simulink model "labFinal_6"  (R2018b)
settings: Solver=FixedStepDiscrete  StartTime=0.0  StopTime=10.0  FixedStep=1  RelTol=1e-3
libraries: hdlsllib x49
settings Model: Creator=mllax8  LastModifiedBy=mllax8

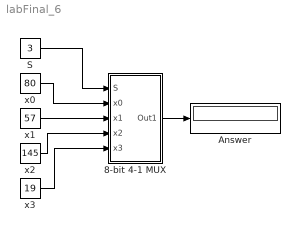
== system labFinal_6 ==
  8-bit 4-1 MUX : Subsystem
  Answer : Display
  S : Constant  Value=3  OutDataTypeStr=uint8  SampleTime=1
  x0 : Constant  Value=80  OutDataTypeStr=uint8  SampleTime=1
  x1 : Constant  Value=57  OutDataTypeStr=uint8  SampleTime=1
  x2 : Constant  Value=145  OutDataTypeStr=uint8  SampleTime=1
  x3 : Constant  Value=19  OutDataTypeStr=uint8  SampleTime=1
  wires:
  x0/1 -> 8-bit 4-1 MUX/2(x0)
  x1/1 -> 8-bit 4-1 MUX/3(x1)
  x2/1 -> 8-bit 4-1 MUX/4(x2)
  x3/1 -> 8-bit 4-1 MUX/5(x3)
  8-bit 4-1 MUX/1(Out1) -> Answer/1
  S/1 -> 8-bit 4-1 MUX/1(S)

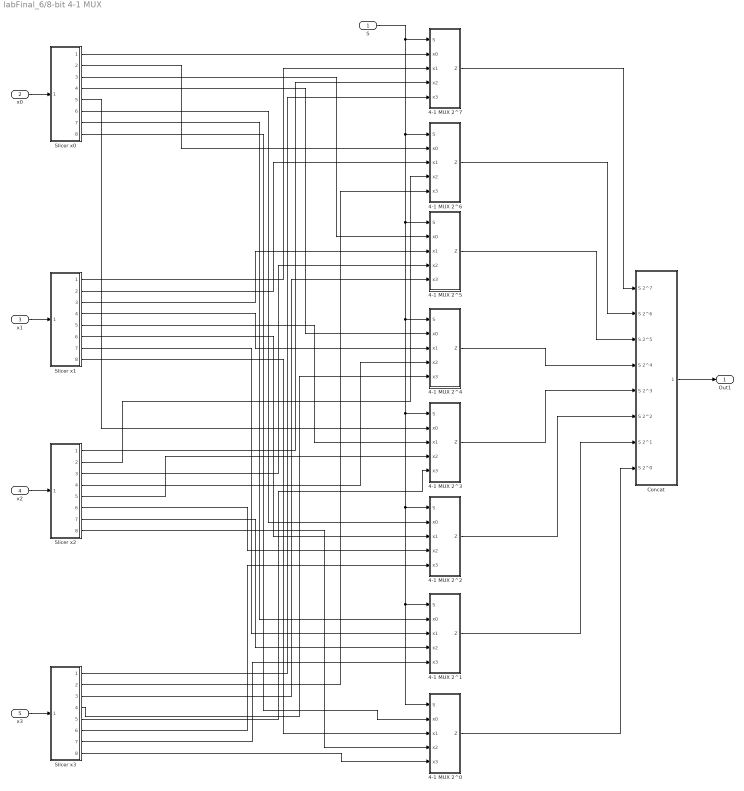
== system labFinal_6/8-bit 4-1 MUX ==
  S : Inport
  x0 : Inport  Port=2
  x1 : Inport  Port=3
  x2 : Inport  Port=4
  x3 : Inport  Port=5
  4-1 MUX 2^0 : Subsystem
  4-1 MUX 2^1 : Subsystem
  4-1 MUX 2^2 : Subsystem
  4-1 MUX 2^3 : Subsystem
  4-1 MUX 2^4 : Subsystem
  4-1 MUX 2^5 : Subsystem
  4-1 MUX 2^6 : Subsystem
  4-1 MUX 2^7 : Subsystem
  Concat : Subsystem
  Slicer x0 : Subsystem
  Slicer x1 : Subsystem
  Slicer x2 : Subsystem
  Slicer x3 : Subsystem
  Out1 : Outport
  wires:
  x1/1 -> Slicer x1/1(uint8)
  x0/1 -> Slicer x0/1(uint8)
  4-1 MUX 2^0/1(Z) -> Concat/8(S 2^0)
  Slicer x2/2(B 2^6) -> 4-1 MUX 2^6/4(x2)
  4-1 MUX 2^2/1(Z) -> Concat/6(S 2^2)
  Slicer x2/7(B 2^1) -> 4-1 MUX 2^1/4(x2)
  4-1 MUX 2^5/1(Z) -> Concat/3(S 2^5)
  Slicer x1/3(B 2^5) -> 4-1 MUX 2^5/3(x1)
  Slicer x0/3(B 2^5) -> 4-1 MUX 2^5/2(x0)
  Slicer x3/8("B 2^0 ") -> 4-1 MUX 2^0/5(x3)
  4-1 MUX 2^4/1(Z) -> Concat/4(S 2^4)
  Slicer x2/8("B 2^0 ") -> 4-1 MUX 2^0/4(x2)
  Slicer x3/1(B 2^7) -> 4-1 MUX 2^7/5(x3)
  Slicer x2/4(B 2^4) -> 4-1 MUX 2^4/4(x2)
  Slicer x0/4(B 2^4) -> 4-1 MUX 2^4/2(x0)
  Slicer x1/8("B 2^0 ") -> 4-1 MUX 2^0/3(x1)
  Slicer x3/4(B 2^4) -> 4-1 MUX 2^4/5(x3)
  4-1 MUX 2^3/1(Z) -> Concat/5(S 2^3)
  Slicer x2/3(B 2^5) -> 4-1 MUX 2^5/4(x2)
  Slicer x3/6(B 2^2) -> 4-1 MUX 2^2/5(x3)
  x3/1 -> Slicer x3/1(uint8)
  Slicer x0/6(B 2^2) -> 4-1 MUX 2^2/2(x0)
  4-1 MUX 2^7/1(Z) -> Concat/1(S 2^7)
  Slicer x1/6(B 2^2) -> 4-1 MUX 2^2/3(x1)
  Slicer x3/2(B 2^6) -> 4-1 MUX 2^6/5(x3)
  Slicer x0/7(B 2^1) -> 4-1 MUX 2^1/2(x0)
  Slicer x2/6(B 2^2) -> 4-1 MUX 2^2/4(x2)
  Slicer x3/3(B 2^5) -> 4-1 MUX 2^5/5(x3)
  Slicer x1/7(B 2^1) -> 4-1 MUX 2^1/3(x1)
  x2/1 -> Slicer x2/1(uint8)
  Slicer x0/5(B 2^3) -> 4-1 MUX 2^3/2(x0)
  Slicer x1/5(B 2^3) -> 4-1 MUX 2^3/3(x1)
  Concat/1(unsign Int) -> Out1/1
  Slicer x2/1(B 2^7) -> 4-1 MUX 2^7/4(x2)
  Slicer x0/8("B 2^0 ") -> 4-1 MUX 2^0/2(x0)
  Slicer x2/5(B 2^3) -> 4-1 MUX 2^3/4(x2)
  4-1 MUX 2^1/1(Z) -> Concat/7(S 2^1)
  Slicer x3/7(B 2^1) -> 4-1 MUX 2^1/5(x3)
  4-1 MUX 2^6/1(Z) -> Concat/2(S 2^6)
  Slicer x1/2(B 2^6) -> 4-1 MUX 2^6/3(x1)
  Slicer x1/4(B 2^4) -> 4-1 MUX 2^4/3(x1)
  Slicer x0/2(B 2^6) -> 4-1 MUX 2^6/2(x0)
  Slicer x3/5(B 2^3) -> 4-1 MUX 2^3/5(x3)
  Slicer x1/1(B 2^7) -> 4-1 MUX 2^7/3(x1)
  S/1 -> 4-1 MUX 2^6/1(S), 4-1 MUX 2^5/1(S), 4-1 MUX 2^4/1(S), 4-1 MUX 2^3/1(S), 4-1 MUX 2^2/1(S), 4-1 MUX 2^0/1(S), 4-1 MUX 2^1/1(S), 4-1 MUX 2^7/1(S)
  Slicer x0/1(B 2^7) -> 4-1 MUX 2^7/2(x0)

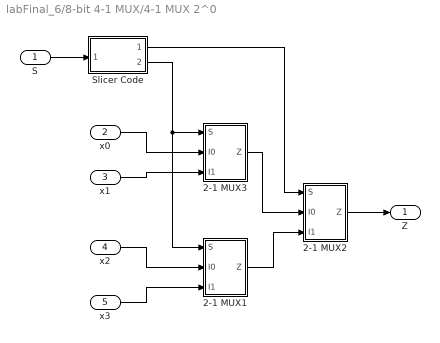
== system labFinal_6/8-bit 4-1 MUX/4-1 MUX 2^0 ==
  S : Inport  OutDataTypeStr=uint8
  x0 : Inport  Port=2  OutDataTypeStr=boolean
  x1 : Inport  Port=3  OutDataTypeStr=boolean
  x2 : Inport  Port=4  OutDataTypeStr=boolean
  x3 : Inport  Port=5  OutDataTypeStr=boolean
  2-1 MUX1 : Subsystem
  2-1 MUX2 : Subsystem
  2-1 MUX3 : Subsystem
  Slicer Code : Subsystem
  Z : Outport
  wires:
  Slicer Code/2("S 2^0 ") -> 2-1 MUX3/1(S), 2-1 MUX1/1(S)
  x0/1 -> 2-1 MUX3/2(I0)
  x1/1 -> 2-1 MUX3/3(I1)
  x2/1 -> 2-1 MUX1/2(I0)
  x3/1 -> 2-1 MUX1/3(I1)
  2-1 MUX3/1(Z) -> 2-1 MUX2/2(I0)
  2-1 MUX1/1(Z) -> 2-1 MUX2/3(I1)
  2-1 MUX2/1(Z) -> Z/1
  S/1 -> Slicer Code/1(uint8)
  Slicer Code/1(S 2^1) -> 2-1 MUX2/1(S)

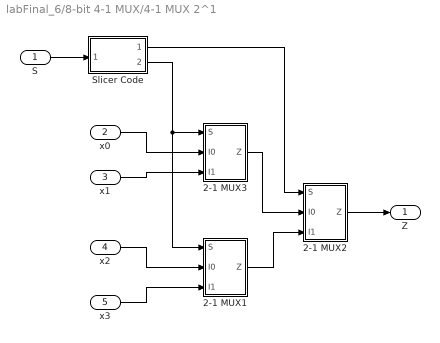
== system labFinal_6/8-bit 4-1 MUX/4-1 MUX 2^1 ==
  S : Inport  OutDataTypeStr=uint8
  x0 : Inport  Port=2  OutDataTypeStr=boolean
  x1 : Inport  Port=3  OutDataTypeStr=boolean
  x2 : Inport  Port=4  OutDataTypeStr=boolean
  x3 : Inport  Port=5  OutDataTypeStr=boolean
  2-1 MUX1 : Subsystem
  2-1 MUX2 : Subsystem
  2-1 MUX3 : Subsystem
  Slicer Code : Subsystem
  Z : Outport
  wires:
  Slicer Code/2("S 2^0 ") -> 2-1 MUX3/1(S), 2-1 MUX1/1(S)
  x0/1 -> 2-1 MUX3/2(I0)
  x1/1 -> 2-1 MUX3/3(I1)
  x2/1 -> 2-1 MUX1/2(I0)
  x3/1 -> 2-1 MUX1/3(I1)
  2-1 MUX3/1(Z) -> 2-1 MUX2/2(I0)
  2-1 MUX1/1(Z) -> 2-1 MUX2/3(I1)
  2-1 MUX2/1(Z) -> Z/1
  S/1 -> Slicer Code/1(uint8)
  Slicer Code/1(S 2^1) -> 2-1 MUX2/1(S)

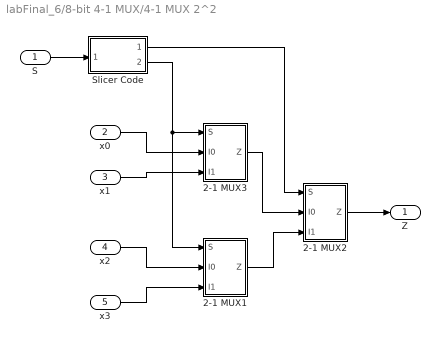
== system labFinal_6/8-bit 4-1 MUX/4-1 MUX 2^2 ==
  S : Inport  OutDataTypeStr=uint8
  x0 : Inport  Port=2  OutDataTypeStr=boolean
  x1 : Inport  Port=3  OutDataTypeStr=boolean
  x2 : Inport  Port=4  OutDataTypeStr=boolean
  x3 : Inport  Port=5  OutDataTypeStr=boolean
  2-1 MUX1 : Subsystem
  2-1 MUX2 : Subsystem
  2-1 MUX3 : Subsystem
  Slicer Code : Subsystem
  Z : Outport
  wires:
  Slicer Code/2("S 2^0 ") -> 2-1 MUX3/1(S), 2-1 MUX1/1(S)
  x0/1 -> 2-1 MUX3/2(I0)
  x1/1 -> 2-1 MUX3/3(I1)
  x2/1 -> 2-1 MUX1/2(I0)
  x3/1 -> 2-1 MUX1/3(I1)
  2-1 MUX3/1(Z) -> 2-1 MUX2/2(I0)
  2-1 MUX1/1(Z) -> 2-1 MUX2/3(I1)
  2-1 MUX2/1(Z) -> Z/1
  S/1 -> Slicer Code/1(uint8)
  Slicer Code/1(S 2^1) -> 2-1 MUX2/1(S)

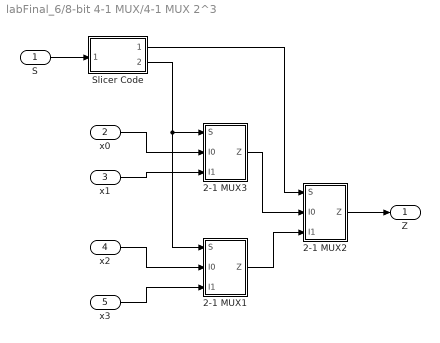
== system labFinal_6/8-bit 4-1 MUX/4-1 MUX 2^3 ==
  S : Inport  OutDataTypeStr=uint8
  x0 : Inport  Port=2  OutDataTypeStr=boolean
  x1 : Inport  Port=3  OutDataTypeStr=boolean
  x2 : Inport  Port=4  OutDataTypeStr=boolean
  x3 : Inport  Port=5  OutDataTypeStr=boolean
  2-1 MUX1 : Subsystem
  2-1 MUX2 : Subsystem
  2-1 MUX3 : Subsystem
  Slicer Code : Subsystem
  Z : Outport
  wires:
  Slicer Code/2("S 2^0 ") -> 2-1 MUX3/1(S), 2-1 MUX1/1(S)
  x0/1 -> 2-1 MUX3/2(I0)
  x1/1 -> 2-1 MUX3/3(I1)
  x2/1 -> 2-1 MUX1/2(I0)
  x3/1 -> 2-1 MUX1/3(I1)
  2-1 MUX3/1(Z) -> 2-1 MUX2/2(I0)
  2-1 MUX1/1(Z) -> 2-1 MUX2/3(I1)
  2-1 MUX2/1(Z) -> Z/1
  S/1 -> Slicer Code/1(uint8)
  Slicer Code/1(S 2^1) -> 2-1 MUX2/1(S)

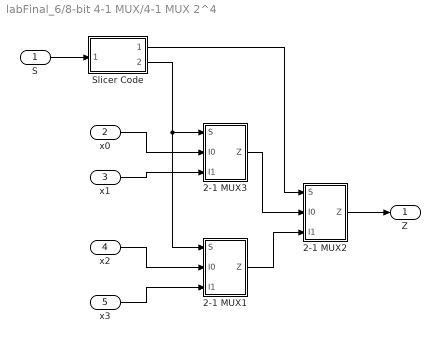
== system labFinal_6/8-bit 4-1 MUX/4-1 MUX 2^4 ==
  S : Inport  OutDataTypeStr=uint8
  x0 : Inport  Port=2  OutDataTypeStr=boolean
  x1 : Inport  Port=3  OutDataTypeStr=boolean
  x2 : Inport  Port=4  OutDataTypeStr=boolean
  x3 : Inport  Port=5  OutDataTypeStr=boolean
  2-1 MUX1 : Subsystem
  2-1 MUX2 : Subsystem
  2-1 MUX3 : Subsystem
  Slicer Code : Subsystem
  Z : Outport
  wires:
  Slicer Code/2("S 2^0 ") -> 2-1 MUX3/1(S), 2-1 MUX1/1(S)
  x0/1 -> 2-1 MUX3/2(I0)
  x1/1 -> 2-1 MUX3/3(I1)
  x2/1 -> 2-1 MUX1/2(I0)
  x3/1 -> 2-1 MUX1/3(I1)
  2-1 MUX3/1(Z) -> 2-1 MUX2/2(I0)
  2-1 MUX1/1(Z) -> 2-1 MUX2/3(I1)
  2-1 MUX2/1(Z) -> Z/1
  S/1 -> Slicer Code/1(uint8)
  Slicer Code/1(S 2^1) -> 2-1 MUX2/1(S)

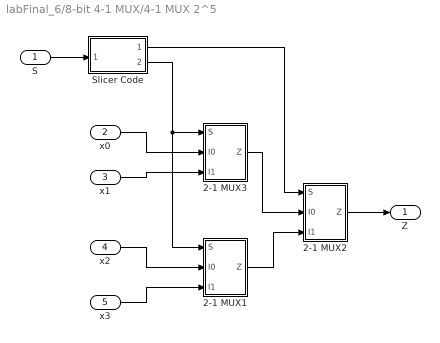
== system labFinal_6/8-bit 4-1 MUX/4-1 MUX 2^5 ==
  S : Inport  OutDataTypeStr=uint8
  x0 : Inport  Port=2  OutDataTypeStr=boolean
  x1 : Inport  Port=3  OutDataTypeStr=boolean
  x2 : Inport  Port=4  OutDataTypeStr=boolean
  x3 : Inport  Port=5  OutDataTypeStr=boolean
  2-1 MUX1 : Subsystem
  2-1 MUX2 : Subsystem
  2-1 MUX3 : Subsystem
  Slicer Code : Subsystem
  Z : Outport
  wires:
  Slicer Code/2("S 2^0 ") -> 2-1 MUX3/1(S), 2-1 MUX1/1(S)
  x0/1 -> 2-1 MUX3/2(I0)
  x1/1 -> 2-1 MUX3/3(I1)
  x2/1 -> 2-1 MUX1/2(I0)
  x3/1 -> 2-1 MUX1/3(I1)
  2-1 MUX3/1(Z) -> 2-1 MUX2/2(I0)
  2-1 MUX1/1(Z) -> 2-1 MUX2/3(I1)
  2-1 MUX2/1(Z) -> Z/1
  S/1 -> Slicer Code/1(uint8)
  Slicer Code/1(S 2^1) -> 2-1 MUX2/1(S)

== system labFinal_6/8-bit 4-1 MUX/4-1 MUX 2^6 ==
  S : Inport  OutDataTypeStr=uint8
  x0 : Inport  Port=2  OutDataTypeStr=boolean
  x1 : Inport  Port=3  OutDataTypeStr=boolean
  x2 : Inport  Port=4  OutDataTypeStr=boolean
  x3 : Inport  Port=5  OutDataTypeStr=boolean
  2-1 MUX1 : Subsystem
  2-1 MUX2 : Subsystem
  2-1 MUX3 : Subsystem
  Slicer Code : Subsystem
  Z : Outport
  wires:
  Slicer Code/2("S 2^0 ") -> 2-1 MUX3/1(S), 2-1 MUX1/1(S)
  x0/1 -> 2-1 MUX3/2(I0)
  x1/1 -> 2-1 MUX3/3(I1)
  x2/1 -> 2-1 MUX1/2(I0)
  x3/1 -> 2-1 MUX1/3(I1)
  2-1 MUX3/1(Z) -> 2-1 MUX2/2(I0)
  2-1 MUX1/1(Z) -> 2-1 MUX2/3(I1)
  2-1 MUX2/1(Z) -> Z/1
  S/1 -> Slicer Code/1(uint8)
  Slicer Code/1(S 2^1) -> 2-1 MUX2/1(S)

== system labFinal_6/8-bit 4-1 MUX/4-1 MUX 2^7 ==
  S : Inport  OutDataTypeStr=uint8
  x0 : Inport  Port=2  OutDataTypeStr=boolean
  x1 : Inport  Port=3  OutDataTypeStr=boolean
  x2 : Inport  Port=4  OutDataTypeStr=boolean
  x3 : Inport  Port=5  OutDataTypeStr=boolean
  2-1 MUX1 : Subsystem
  2-1 MUX2 : Subsystem
  2-1 MUX3 : Subsystem
  Slicer Code : Subsystem
  Z : Outport
  wires:
  Slicer Code/2("S 2^0 ") -> 2-1 MUX3/1(S), 2-1 MUX1/1(S)
  x0/1 -> 2-1 MUX3/2(I0)
  x1/1 -> 2-1 MUX3/3(I1)
  x2/1 -> 2-1 MUX1/2(I0)
  x3/1 -> 2-1 MUX1/3(I1)
  2-1 MUX3/1(Z) -> 2-1 MUX2/2(I0)
  2-1 MUX1/1(Z) -> 2-1 MUX2/3(I1)
  2-1 MUX2/1(Z) -> Z/1
  S/1 -> Slicer Code/1(uint8)
  Slicer Code/1(S 2^1) -> 2-1 MUX2/1(S)

== system labFinal_6/8-bit 4-1 MUX/Concat ==
  S 2^7 : Inport
  S 2^6 : Inport  Port=2
  S 2^5 : Inport  Port=3
  S 2^4 : Inport  Port=4
  S 2^3 : Inport  Port=5
  S 2^2 : Inport  Port=6
  S 2^1 : Inport  Port=7
  S 2^0 : Inport  Port=8
  Bit Concat : hdlsllib/Logic and Bit Operations/Bit Concat  numInputs=8
      settings: SourceProductName=HDL Coder  SourceProductBaseCode=HD
  unsign Int : Outport
  wires:
  Bit Concat/1 -> unsign Int/1
  S 2^3/1 -> Bit Concat/5
  S 2^5/1 -> Bit Concat/3
  S 2^4/1 -> Bit Concat/4
  S 2^0/1 -> Bit Concat/8
  S 2^7/1 -> Bit Concat/1
  S 2^1/1 -> Bit Concat/7
  S 2^6/1 -> Bit Concat/2
  S 2^2/1 -> Bit Concat/6

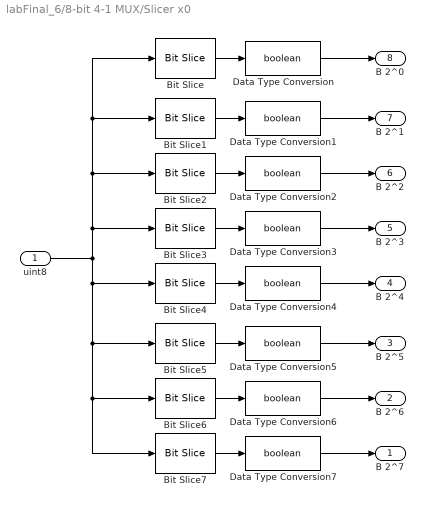
== system labFinal_6/8-bit 4-1 MUX/Slicer x0 ==
  uint8 : Inport  OutDataTypeStr=uint8  SampleTime=1
  Bit Slice : hdlsllib/Logic and Bit Operations/Bit Slice  lidx=0  ridx=0
  Bit Slice1 : hdlsllib/Logic and Bit Operations/Bit Slice  lidx=1  ridx=1
  Bit Slice2 : hdlsllib/Logic and Bit Operations/Bit Slice  lidx=2  ridx=2
  Bit Slice3 : hdlsllib/Logic and Bit Operations/Bit Slice  lidx=3  ridx=3
  Bit Slice4 : hdlsllib/Logic and Bit Operations/Bit Slice  lidx=4  ridx=4
  Bit Slice5 : hdlsllib/Logic and Bit Operations/Bit Slice  lidx=5  ridx=5
  Bit Slice6 : hdlsllib/Logic and Bit Operations/Bit Slice  lidx=6  ridx=6
  Bit Slice7 : hdlsllib/Logic and Bit Operations/Bit Slice  lidx=7  ridx=7
  Data Type Conversion{,1..7} (8 alike) : DataTypeConversion  OutDataTypeStr=boolean
  B 2^7 : Outport
  B 2^6 : Outport  Port=2
  B 2^5 : Outport  Port=3
  B 2^4 : Outport  Port=4
  B 2^3 : Outport  Port=5
  B 2^2 : Outport  Port=6
  B 2^1 : Outport  Port=7
  "B 2^0 " : Outport  Port=8
  wires:
  Data Type Conversion/1 -> "B 2^0 "/1
  Data Type Conversion5/1 -> B 2^5/1
  Bit Slice1/1 -> Data Type Conversion1/1
  Bit Slice5/1 -> Data Type Conversion5/1
  Bit Slice7/1 -> Data Type Conversion7/1
  Bit Slice2/1 -> Data Type Conversion2/1
  Bit Slice3/1 -> Data Type Conversion3/1
  Data Type Conversion6/1 -> B 2^6/1
  Bit Slice4/1 -> Data Type Conversion4/1
  uint8/1 -> Bit Slice4/1, Bit Slice5/1, Bit Slice6/1, Bit Slice7/1, Bit Slice3/1, Bit Slice2/1, Bit Slice1/1, Bit Slice/1
  Data Type Conversion1/1 -> B 2^1/1
  Data Type Conversion2/1 -> B 2^2/1
  Bit Slice/1 -> Data Type Conversion/1
  Bit Slice6/1 -> Data Type Conversion6/1
  Data Type Conversion3/1 -> B 2^3/1
  Data Type Conversion4/1 -> B 2^4/1
  Data Type Conversion7/1 -> B 2^7/1

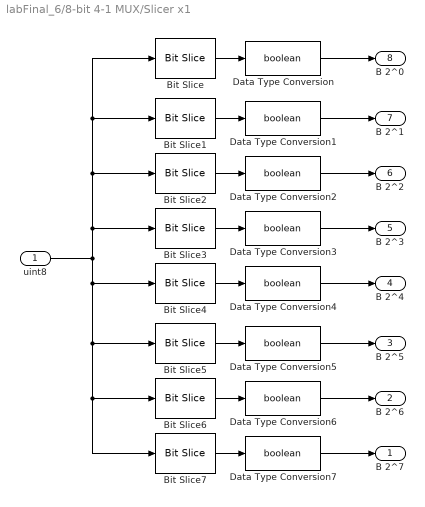
== system labFinal_6/8-bit 4-1 MUX/Slicer x1 ==
  uint8 : Inport  OutDataTypeStr=uint8  SampleTime=1
  Bit Slice : hdlsllib/Logic and Bit Operations/Bit Slice  lidx=0  ridx=0
  Bit Slice1 : hdlsllib/Logic and Bit Operations/Bit Slice  lidx=1  ridx=1
  Bit Slice2 : hdlsllib/Logic and Bit Operations/Bit Slice  lidx=2  ridx=2
  Bit Slice3 : hdlsllib/Logic and Bit Operations/Bit Slice  lidx=3  ridx=3
  Bit Slice4 : hdlsllib/Logic and Bit Operations/Bit Slice  lidx=4  ridx=4
  Bit Slice5 : hdlsllib/Logic and Bit Operations/Bit Slice  lidx=5  ridx=5
  Bit Slice6 : hdlsllib/Logic and Bit Operations/Bit Slice  lidx=6  ridx=6
  Bit Slice7 : hdlsllib/Logic and Bit Operations/Bit Slice  lidx=7  ridx=7
  Data Type Conversion{,1..7} (8 alike) : DataTypeConversion  OutDataTypeStr=boolean
  B 2^7 : Outport
  B 2^6 : Outport  Port=2
  B 2^5 : Outport  Port=3
  B 2^4 : Outport  Port=4
  B 2^3 : Outport  Port=5
  B 2^2 : Outport  Port=6
  B 2^1 : Outport  Port=7
  "B 2^0 " : Outport  Port=8
  wires:
  Data Type Conversion/1 -> "B 2^0 "/1
  Data Type Conversion5/1 -> B 2^5/1
  Bit Slice1/1 -> Data Type Conversion1/1
  Bit Slice5/1 -> Data Type Conversion5/1
  Bit Slice7/1 -> Data Type Conversion7/1
  Bit Slice2/1 -> Data Type Conversion2/1
  Bit Slice3/1 -> Data Type Conversion3/1
  Data Type Conversion6/1 -> B 2^6/1
  Bit Slice4/1 -> Data Type Conversion4/1
  uint8/1 -> Bit Slice4/1, Bit Slice5/1, Bit Slice6/1, Bit Slice7/1, Bit Slice3/1, Bit Slice2/1, Bit Slice1/1, Bit Slice/1
  Data Type Conversion1/1 -> B 2^1/1
  Data Type Conversion2/1 -> B 2^2/1
  Bit Slice/1 -> Data Type Conversion/1
  Bit Slice6/1 -> Data Type Conversion6/1
  Data Type Conversion3/1 -> B 2^3/1
  Data Type Conversion4/1 -> B 2^4/1
  Data Type Conversion7/1 -> B 2^7/1

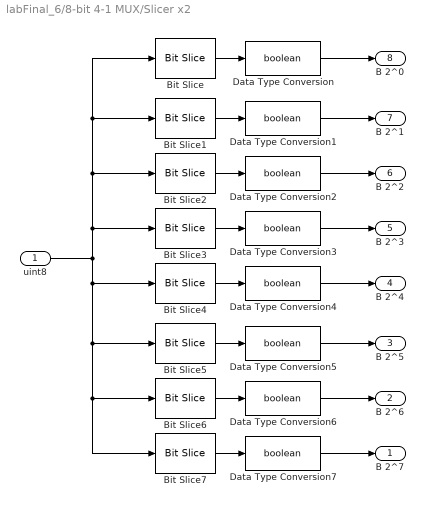
== system labFinal_6/8-bit 4-1 MUX/Slicer x2 ==
  uint8 : Inport  OutDataTypeStr=uint8  SampleTime=1
  Bit Slice : hdlsllib/Logic and Bit Operations/Bit Slice  lidx=0  ridx=0
  Bit Slice1 : hdlsllib/Logic and Bit Operations/Bit Slice  lidx=1  ridx=1
  Bit Slice2 : hdlsllib/Logic and Bit Operations/Bit Slice  lidx=2  ridx=2
  Bit Slice3 : hdlsllib/Logic and Bit Operations/Bit Slice  lidx=3  ridx=3
  Bit Slice4 : hdlsllib/Logic and Bit Operations/Bit Slice  lidx=4  ridx=4
  Bit Slice5 : hdlsllib/Logic and Bit Operations/Bit Slice  lidx=5  ridx=5
  Bit Slice6 : hdlsllib/Logic and Bit Operations/Bit Slice  lidx=6  ridx=6
  Bit Slice7 : hdlsllib/Logic and Bit Operations/Bit Slice  lidx=7  ridx=7
  Data Type Conversion{,1..7} (8 alike) : DataTypeConversion  OutDataTypeStr=boolean
  B 2^7 : Outport
  B 2^6 : Outport  Port=2
  B 2^5 : Outport  Port=3
  B 2^4 : Outport  Port=4
  B 2^3 : Outport  Port=5
  B 2^2 : Outport  Port=6
  B 2^1 : Outport  Port=7
  "B 2^0 " : Outport  Port=8
  wires:
  Data Type Conversion/1 -> "B 2^0 "/1
  Data Type Conversion5/1 -> B 2^5/1
  Bit Slice1/1 -> Data Type Conversion1/1
  Bit Slice5/1 -> Data Type Conversion5/1
  Bit Slice7/1 -> Data Type Conversion7/1
  Bit Slice2/1 -> Data Type Conversion2/1
  Bit Slice3/1 -> Data Type Conversion3/1
  Data Type Conversion6/1 -> B 2^6/1
  Bit Slice4/1 -> Data Type Conversion4/1
  uint8/1 -> Bit Slice4/1, Bit Slice5/1, Bit Slice6/1, Bit Slice7/1, Bit Slice3/1, Bit Slice2/1, Bit Slice1/1, Bit Slice/1
  Data Type Conversion1/1 -> B 2^1/1
  Data Type Conversion2/1 -> B 2^2/1
  Bit Slice/1 -> Data Type Conversion/1
  Bit Slice6/1 -> Data Type Conversion6/1
  Data Type Conversion3/1 -> B 2^3/1
  Data Type Conversion4/1 -> B 2^4/1
  Data Type Conversion7/1 -> B 2^7/1

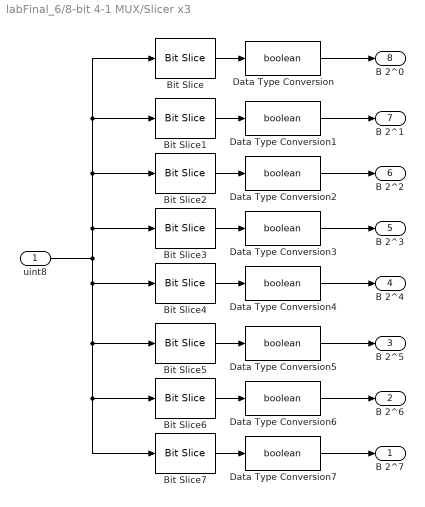
== system labFinal_6/8-bit 4-1 MUX/Slicer x3 ==
  uint8 : Inport  OutDataTypeStr=uint8  SampleTime=1
  Bit Slice : hdlsllib/Logic and Bit Operations/Bit Slice  lidx=0  ridx=0
  Bit Slice1 : hdlsllib/Logic and Bit Operations/Bit Slice  lidx=1  ridx=1
  Bit Slice2 : hdlsllib/Logic and Bit Operations/Bit Slice  lidx=2  ridx=2
  Bit Slice3 : hdlsllib/Logic and Bit Operations/Bit Slice  lidx=3  ridx=3
  Bit Slice4 : hdlsllib/Logic and Bit Operations/Bit Slice  lidx=4  ridx=4
  Bit Slice5 : hdlsllib/Logic and Bit Operations/Bit Slice  lidx=5  ridx=5
  Bit Slice6 : hdlsllib/Logic and Bit Operations/Bit Slice  lidx=6  ridx=6
  Bit Slice7 : hdlsllib/Logic and Bit Operations/Bit Slice  lidx=7  ridx=7
  Data Type Conversion{,1..7} (8 alike) : DataTypeConversion  OutDataTypeStr=boolean
  B 2^7 : Outport
  B 2^6 : Outport  Port=2
  B 2^5 : Outport  Port=3
  B 2^4 : Outport  Port=4
  B 2^3 : Outport  Port=5
  B 2^2 : Outport  Port=6
  B 2^1 : Outport  Port=7
  "B 2^0 " : Outport  Port=8
  wires:
  Data Type Conversion/1 -> "B 2^0 "/1
  Data Type Conversion5/1 -> B 2^5/1
  Bit Slice1/1 -> Data Type Conversion1/1
  Bit Slice5/1 -> Data Type Conversion5/1
  Bit Slice7/1 -> Data Type Conversion7/1
  Bit Slice2/1 -> Data Type Conversion2/1
  Bit Slice3/1 -> Data Type Conversion3/1
  Data Type Conversion6/1 -> B 2^6/1
  Bit Slice4/1 -> Data Type Conversion4/1
  uint8/1 -> Bit Slice4/1, Bit Slice5/1, Bit Slice6/1, Bit Slice7/1, Bit Slice3/1, Bit Slice2/1, Bit Slice1/1, Bit Slice/1
  Data Type Conversion1/1 -> B 2^1/1
  Data Type Conversion2/1 -> B 2^2/1
  Bit Slice/1 -> Data Type Conversion/1
  Bit Slice6/1 -> Data Type Conversion6/1
  Data Type Conversion3/1 -> B 2^3/1
  Data Type Conversion4/1 -> B 2^4/1
  Data Type Conversion7/1 -> B 2^7/1

== system labFinal_6/8-bit 4-1 MUX/4-1 MUX 2^0/2-1 MUX1 ==
  S : Inport
  I0 : Inport  Port=2
  I1 : Inport  Port=3
  Data Type Conversion1 : DataTypeConversion  OutDataTypeStr=boolean
  Data Type Conversion2 : DataTypeConversion  OutDataTypeStr=boolean
  Logical Operator : Logic  AllPortsSameDT=off  OutDataTypeStr=boolean
  Logical Operator1 : Logic  AllPortsSameDT=off  OutDataTypeStr=boolean
  Logical Operator2 : Logic  Operator=OR  AllPortsSameDT=off  OutDataTypeStr=boolean
  Logical Operator3 : Logic  Operator=NOT  AllPortsSameDT=off  OutDataTypeStr=boolean
  Z : Outport
  wires:
  Logical Operator2/1 -> Z/1
  I1/1 -> Data Type Conversion2/1
  Logical Operator1/1 -> Logical Operator2/2
  S/1 -> Logical Operator3/1, Logical Operator1/1
  I0/1 -> Data Type Conversion1/1
  Logical Operator/1 -> Logical Operator2/1
  Data Type Conversion1/1 -> Logical Operator/1
  Data Type Conversion2/1 -> Logical Operator1/2
  Logical Operator3/1 -> Logical Operator/2

== system labFinal_6/8-bit 4-1 MUX/4-1 MUX 2^0/2-1 MUX2 ==
  S : Inport
  I0 : Inport  Port=2
  I1 : Inport  Port=3
  Data Type Conversion1 : DataTypeConversion  OutDataTypeStr=boolean
  Data Type Conversion2 : DataTypeConversion  OutDataTypeStr=boolean
  Logical Operator : Logic  AllPortsSameDT=off  OutDataTypeStr=boolean
  Logical Operator1 : Logic  AllPortsSameDT=off  OutDataTypeStr=boolean
  Logical Operator2 : Logic  Operator=OR  AllPortsSameDT=off  OutDataTypeStr=boolean
  Logical Operator3 : Logic  Operator=NOT  AllPortsSameDT=off  OutDataTypeStr=boolean
  Z : Outport
  wires:
  Logical Operator2/1 -> Z/1
  I1/1 -> Data Type Conversion2/1
  Logical Operator1/1 -> Logical Operator2/2
  S/1 -> Logical Operator3/1, Logical Operator1/1
  I0/1 -> Data Type Conversion1/1
  Logical Operator/1 -> Logical Operator2/1
  Data Type Conversion1/1 -> Logical Operator/1
  Data Type Conversion2/1 -> Logical Operator1/2
  Logical Operator3/1 -> Logical Operator/2

== system labFinal_6/8-bit 4-1 MUX/4-1 MUX 2^0/2-1 MUX3 ==
  S : Inport
  I0 : Inport  Port=2
  I1 : Inport  Port=3
  Data Type Conversion1 : DataTypeConversion  OutDataTypeStr=boolean
  Data Type Conversion2 : DataTypeConversion  OutDataTypeStr=boolean
  Logical Operator : Logic  AllPortsSameDT=off  OutDataTypeStr=boolean
  Logical Operator1 : Logic  AllPortsSameDT=off  OutDataTypeStr=boolean
  Logical Operator2 : Logic  Operator=OR  AllPortsSameDT=off  OutDataTypeStr=boolean
  Logical Operator3 : Logic  Operator=NOT  AllPortsSameDT=off  OutDataTypeStr=boolean
  Z : Outport
  wires:
  Logical Operator2/1 -> Z/1
  I1/1 -> Data Type Conversion2/1
  Logical Operator1/1 -> Logical Operator2/2
  S/1 -> Logical Operator3/1, Logical Operator1/1
  I0/1 -> Data Type Conversion1/1
  Logical Operator/1 -> Logical Operator2/1
  Data Type Conversion1/1 -> Logical Operator/1
  Data Type Conversion2/1 -> Logical Operator1/2
  Logical Operator3/1 -> Logical Operator/2

== system labFinal_6/8-bit 4-1 MUX/4-1 MUX 2^0/Slicer Code ==
  uint8 : Inport  OutDataTypeStr=uint8  SampleTime=1
  Bit Slice : hdlsllib/Logic and Bit Operations/Bit Slice  lidx=0  ridx=0
  Bit Slice1 : hdlsllib/Logic and Bit Operations/Bit Slice  lidx=1  ridx=1
  Data Type Conversion : DataTypeConversion  OutDataTypeStr=boolean
  Data Type Conversion1 : DataTypeConversion  OutDataTypeStr=boolean
  S 2^1 : Outport
  "S 2^0 " : Outport  Port=2
  wires:
  Data Type Conversion1/1 -> S 2^1/1
  Data Type Conversion/1 -> "S 2^0 "/1
  Bit Slice1/1 -> Data Type Conversion1/1
  Bit Slice/1 -> Data Type Conversion/1
  uint8/1 -> Bit Slice/1, Bit Slice1/1

== system labFinal_6/8-bit 4-1 MUX/4-1 MUX 2^1/2-1 MUX1 ==
  S : Inport
  I0 : Inport  Port=2
  I1 : Inport  Port=3
  Data Type Conversion1 : DataTypeConversion  OutDataTypeStr=boolean
  Data Type Conversion2 : DataTypeConversion  OutDataTypeStr=boolean
  Logical Operator : Logic  AllPortsSameDT=off  OutDataTypeStr=boolean
  Logical Operator1 : Logic  AllPortsSameDT=off  OutDataTypeStr=boolean
  Logical Operator2 : Logic  Operator=OR  AllPortsSameDT=off  OutDataTypeStr=boolean
  Logical Operator3 : Logic  Operator=NOT  AllPortsSameDT=off  OutDataTypeStr=boolean
  Z : Outport
  wires:
  Logical Operator2/1 -> Z/1
  I1/1 -> Data Type Conversion2/1
  Logical Operator1/1 -> Logical Operator2/2
  S/1 -> Logical Operator3/1, Logical Operator1/1
  I0/1 -> Data Type Conversion1/1
  Logical Operator/1 -> Logical Operator2/1
  Data Type Conversion1/1 -> Logical Operator/1
  Data Type Conversion2/1 -> Logical Operator1/2
  Logical Operator3/1 -> Logical Operator/2

== system labFinal_6/8-bit 4-1 MUX/4-1 MUX 2^1/2-1 MUX2 ==
  S : Inport
  I0 : Inport  Port=2
  I1 : Inport  Port=3
  Data Type Conversion1 : DataTypeConversion  OutDataTypeStr=boolean
  Data Type Conversion2 : DataTypeConversion  OutDataTypeStr=boolean
  Logical Operator : Logic  AllPortsSameDT=off  OutDataTypeStr=boolean
  Logical Operator1 : Logic  AllPortsSameDT=off  OutDataTypeStr=boolean
  Logical Operator2 : Logic  Operator=OR  AllPortsSameDT=off  OutDataTypeStr=boolean
  Logical Operator3 : Logic  Operator=NOT  AllPortsSameDT=off  OutDataTypeStr=boolean
  Z : Outport
  wires:
  Logical Operator2/1 -> Z/1
  I1/1 -> Data Type Conversion2/1
  Logical Operator1/1 -> Logical Operator2/2
  S/1 -> Logical Operator3/1, Logical Operator1/1
  I0/1 -> Data Type Conversion1/1
  Logical Operator/1 -> Logical Operator2/1
  Data Type Conversion1/1 -> Logical Operator/1
  Data Type Conversion2/1 -> Logical Operator1/2
  Logical Operator3/1 -> Logical Operator/2

== system labFinal_6/8-bit 4-1 MUX/4-1 MUX 2^1/2-1 MUX3 ==
  S : Inport
  I0 : Inport  Port=2
  I1 : Inport  Port=3
  Data Type Conversion1 : DataTypeConversion  OutDataTypeStr=boolean
  Data Type Conversion2 : DataTypeConversion  OutDataTypeStr=boolean
  Logical Operator : Logic  AllPortsSameDT=off  OutDataTypeStr=boolean
  Logical Operator1 : Logic  AllPortsSameDT=off  OutDataTypeStr=boolean
  Logical Operator2 : Logic  Operator=OR  AllPortsSameDT=off  OutDataTypeStr=boolean
  Logical Operator3 : Logic  Operator=NOT  AllPortsSameDT=off  OutDataTypeStr=boolean
  Z : Outport
  wires:
  Logical Operator2/1 -> Z/1
  I1/1 -> Data Type Conversion2/1
  Logical Operator1/1 -> Logical Operator2/2
  S/1 -> Logical Operator3/1, Logical Operator1/1
  I0/1 -> Data Type Conversion1/1
  Logical Operator/1 -> Logical Operator2/1
  Data Type Conversion1/1 -> Logical Operator/1
  Data Type Conversion2/1 -> Logical Operator1/2
  Logical Operator3/1 -> Logical Operator/2

== system labFinal_6/8-bit 4-1 MUX/4-1 MUX 2^1/Slicer Code ==
  uint8 : Inport  OutDataTypeStr=uint8  SampleTime=1
  Bit Slice : hdlsllib/Logic and Bit Operations/Bit Slice  lidx=0  ridx=0
  Bit Slice1 : hdlsllib/Logic and Bit Operations/Bit Slice  lidx=1  ridx=1
  Data Type Conversion : DataTypeConversion  OutDataTypeStr=boolean
  Data Type Conversion1 : DataTypeConversion  OutDataTypeStr=boolean
  S 2^1 : Outport
  "S 2^0 " : Outport  Port=2
  wires:
  Data Type Conversion1/1 -> S 2^1/1
  Data Type Conversion/1 -> "S 2^0 "/1
  Bit Slice1/1 -> Data Type Conversion1/1
  Bit Slice/1 -> Data Type Conversion/1
  uint8/1 -> Bit Slice/1, Bit Slice1/1

== system labFinal_6/8-bit 4-1 MUX/4-1 MUX 2^2/2-1 MUX1 ==
  S : Inport
  I0 : Inport  Port=2
  I1 : Inport  Port=3
  Data Type Conversion1 : DataTypeConversion  OutDataTypeStr=boolean
  Data Type Conversion2 : DataTypeConversion  OutDataTypeStr=boolean
  Logical Operator : Logic  AllPortsSameDT=off  OutDataTypeStr=boolean
  Logical Operator1 : Logic  AllPortsSameDT=off  OutDataTypeStr=boolean
  Logical Operator2 : Logic  Operator=OR  AllPortsSameDT=off  OutDataTypeStr=boolean
  Logical Operator3 : Logic  Operator=NOT  AllPortsSameDT=off  OutDataTypeStr=boolean
  Z : Outport
  wires:
  Logical Operator2/1 -> Z/1
  I1/1 -> Data Type Conversion2/1
  Logical Operator1/1 -> Logical Operator2/2
  S/1 -> Logical Operator3/1, Logical Operator1/1
  I0/1 -> Data Type Conversion1/1
  Logical Operator/1 -> Logical Operator2/1
  Data Type Conversion1/1 -> Logical Operator/1
  Data Type Conversion2/1 -> Logical Operator1/2
  Logical Operator3/1 -> Logical Operator/2

== system labFinal_6/8-bit 4-1 MUX/4-1 MUX 2^2/2-1 MUX2 ==
  S : Inport
  I0 : Inport  Port=2
  I1 : Inport  Port=3
  Data Type Conversion1 : DataTypeConversion  OutDataTypeStr=boolean
  Data Type Conversion2 : DataTypeConversion  OutDataTypeStr=boolean
  Logical Operator : Logic  AllPortsSameDT=off  OutDataTypeStr=boolean
  Logical Operator1 : Logic  AllPortsSameDT=off  OutDataTypeStr=boolean
  Logical Operator2 : Logic  Operator=OR  AllPortsSameDT=off  OutDataTypeStr=boolean
  Logical Operator3 : Logic  Operator=NOT  AllPortsSameDT=off  OutDataTypeStr=boolean
  Z : Outport
  wires:
  Logical Operator2/1 -> Z/1
  I1/1 -> Data Type Conversion2/1
  Logical Operator1/1 -> Logical Operator2/2
  S/1 -> Logical Operator3/1, Logical Operator1/1
  I0/1 -> Data Type Conversion1/1
  Logical Operator/1 -> Logical Operator2/1
  Data Type Conversion1/1 -> Logical Operator/1
  Data Type Conversion2/1 -> Logical Operator1/2
  Logical Operator3/1 -> Logical Operator/2

== system labFinal_6/8-bit 4-1 MUX/4-1 MUX 2^2/2-1 MUX3 ==
  S : Inport
  I0 : Inport  Port=2
  I1 : Inport  Port=3
  Data Type Conversion1 : DataTypeConversion  OutDataTypeStr=boolean
  Data Type Conversion2 : DataTypeConversion  OutDataTypeStr=boolean
  Logical Operator : Logic  AllPortsSameDT=off  OutDataTypeStr=boolean
  Logical Operator1 : Logic  AllPortsSameDT=off  OutDataTypeStr=boolean
  Logical Operator2 : Logic  Operator=OR  AllPortsSameDT=off  OutDataTypeStr=boolean
  Logical Operator3 : Logic  Operator=NOT  AllPortsSameDT=off  OutDataTypeStr=boolean
  Z : Outport
  wires:
  Logical Operator2/1 -> Z/1
  I1/1 -> Data Type Conversion2/1
  Logical Operator1/1 -> Logical Operator2/2
  S/1 -> Logical Operator3/1, Logical Operator1/1
  I0/1 -> Data Type Conversion1/1
  Logical Operator/1 -> Logical Operator2/1
  Data Type Conversion1/1 -> Logical Operator/1
  Data Type Conversion2/1 -> Logical Operator1/2
  Logical Operator3/1 -> Logical Operator/2

== system labFinal_6/8-bit 4-1 MUX/4-1 MUX 2^2/Slicer Code ==
  uint8 : Inport  OutDataTypeStr=uint8  SampleTime=1
  Bit Slice : hdlsllib/Logic and Bit Operations/Bit Slice  lidx=0  ridx=0
  Bit Slice1 : hdlsllib/Logic and Bit Operations/Bit Slice  lidx=1  ridx=1
  Data Type Conversion : DataTypeConversion  OutDataTypeStr=boolean
  Data Type Conversion1 : DataTypeConversion  OutDataTypeStr=boolean
  S 2^1 : Outport
  "S 2^0 " : Outport  Port=2
  wires:
  Data Type Conversion1/1 -> S 2^1/1
  Data Type Conversion/1 -> "S 2^0 "/1
  Bit Slice1/1 -> Data Type Conversion1/1
  Bit Slice/1 -> Data Type Conversion/1
  uint8/1 -> Bit Slice/1, Bit Slice1/1

== system labFinal_6/8-bit 4-1 MUX/4-1 MUX 2^3/2-1 MUX1 ==
  S : Inport
  I0 : Inport  Port=2
  I1 : Inport  Port=3
  Data Type Conversion1 : DataTypeConversion  OutDataTypeStr=boolean
  Data Type Conversion2 : DataTypeConversion  OutDataTypeStr=boolean
  Logical Operator : Logic  AllPortsSameDT=off  OutDataTypeStr=boolean
  Logical Operator1 : Logic  AllPortsSameDT=off  OutDataTypeStr=boolean
  Logical Operator2 : Logic  Operator=OR  AllPortsSameDT=off  OutDataTypeStr=boolean
  Logical Operator3 : Logic  Operator=NOT  AllPortsSameDT=off  OutDataTypeStr=boolean
  Z : Outport
  wires:
  Logical Operator2/1 -> Z/1
  I1/1 -> Data Type Conversion2/1
  Logical Operator1/1 -> Logical Operator2/2
  S/1 -> Logical Operator3/1, Logical Operator1/1
  I0/1 -> Data Type Conversion1/1
  Logical Operator/1 -> Logical Operator2/1
  Data Type Conversion1/1 -> Logical Operator/1
  Data Type Conversion2/1 -> Logical Operator1/2
  Logical Operator3/1 -> Logical Operator/2

== system labFinal_6/8-bit 4-1 MUX/4-1 MUX 2^3/2-1 MUX2 ==
  S : Inport
  I0 : Inport  Port=2
  I1 : Inport  Port=3
  Data Type Conversion1 : DataTypeConversion  OutDataTypeStr=boolean
  Data Type Conversion2 : DataTypeConversion  OutDataTypeStr=boolean
  Logical Operator : Logic  AllPortsSameDT=off  OutDataTypeStr=boolean
  Logical Operator1 : Logic  AllPortsSameDT=off  OutDataTypeStr=boolean
  Logical Operator2 : Logic  Operator=OR  AllPortsSameDT=off  OutDataTypeStr=boolean
  Logical Operator3 : Logic  Operator=NOT  AllPortsSameDT=off  OutDataTypeStr=boolean
  Z : Outport
  wires:
  Logical Operator2/1 -> Z/1
  I1/1 -> Data Type Conversion2/1
  Logical Operator1/1 -> Logical Operator2/2
  S/1 -> Logical Operator3/1, Logical Operator1/1
  I0/1 -> Data Type Conversion1/1
  Logical Operator/1 -> Logical Operator2/1
  Data Type Conversion1/1 -> Logical Operator/1
  Data Type Conversion2/1 -> Logical Operator1/2
  Logical Operator3/1 -> Logical Operator/2

== system labFinal_6/8-bit 4-1 MUX/4-1 MUX 2^3/2-1 MUX3 ==
  S : Inport
  I0 : Inport  Port=2
  I1 : Inport  Port=3
  Data Type Conversion1 : DataTypeConversion  OutDataTypeStr=boolean
  Data Type Conversion2 : DataTypeConversion  OutDataTypeStr=boolean
  Logical Operator : Logic  AllPortsSameDT=off  OutDataTypeStr=boolean
  Logical Operator1 : Logic  AllPortsSameDT=off  OutDataTypeStr=boolean
  Logical Operator2 : Logic  Operator=OR  AllPortsSameDT=off  OutDataTypeStr=boolean
  Logical Operator3 : Logic  Operator=NOT  AllPortsSameDT=off  OutDataTypeStr=boolean
  Z : Outport
  wires:
  Logical Operator2/1 -> Z/1
  I1/1 -> Data Type Conversion2/1
  Logical Operator1/1 -> Logical Operator2/2
  S/1 -> Logical Operator3/1, Logical Operator1/1
  I0/1 -> Data Type Conversion1/1
  Logical Operator/1 -> Logical Operator2/1
  Data Type Conversion1/1 -> Logical Operator/1
  Data Type Conversion2/1 -> Logical Operator1/2
  Logical Operator3/1 -> Logical Operator/2

== system labFinal_6/8-bit 4-1 MUX/4-1 MUX 2^3/Slicer Code ==
  uint8 : Inport  OutDataTypeStr=uint8  SampleTime=1
  Bit Slice : hdlsllib/Logic and Bit Operations/Bit Slice  lidx=0  ridx=0
  Bit Slice1 : hdlsllib/Logic and Bit Operations/Bit Slice  lidx=1  ridx=1
  Data Type Conversion : DataTypeConversion  OutDataTypeStr=boolean
  Data Type Conversion1 : DataTypeConversion  OutDataTypeStr=boolean
  S 2^1 : Outport
  "S 2^0 " : Outport  Port=2
  wires:
  Data Type Conversion1/1 -> S 2^1/1
  Data Type Conversion/1 -> "S 2^0 "/1
  Bit Slice1/1 -> Data Type Conversion1/1
  Bit Slice/1 -> Data Type Conversion/1
  uint8/1 -> Bit Slice/1, Bit Slice1/1

== system labFinal_6/8-bit 4-1 MUX/4-1 MUX 2^4/2-1 MUX1 ==
  S : Inport
  I0 : Inport  Port=2
  I1 : Inport  Port=3
  Data Type Conversion1 : DataTypeConversion  OutDataTypeStr=boolean
  Data Type Conversion2 : DataTypeConversion  OutDataTypeStr=boolean
  Logical Operator : Logic  AllPortsSameDT=off  OutDataTypeStr=boolean
  Logical Operator1 : Logic  AllPortsSameDT=off  OutDataTypeStr=boolean
  Logical Operator2 : Logic  Operator=OR  AllPortsSameDT=off  OutDataTypeStr=boolean
  Logical Operator3 : Logic  Operator=NOT  AllPortsSameDT=off  OutDataTypeStr=boolean
  Z : Outport
  wires:
  Logical Operator2/1 -> Z/1
  I1/1 -> Data Type Conversion2/1
  Logical Operator1/1 -> Logical Operator2/2
  S/1 -> Logical Operator3/1, Logical Operator1/1
  I0/1 -> Data Type Conversion1/1
  Logical Operator/1 -> Logical Operator2/1
  Data Type Conversion1/1 -> Logical Operator/1
  Data Type Conversion2/1 -> Logical Operator1/2
  Logical Operator3/1 -> Logical Operator/2

== system labFinal_6/8-bit 4-1 MUX/4-1 MUX 2^4/2-1 MUX2 ==
  S : Inport
  I0 : Inport  Port=2
  I1 : Inport  Port=3
  Data Type Conversion1 : DataTypeConversion  OutDataTypeStr=boolean
  Data Type Conversion2 : DataTypeConversion  OutDataTypeStr=boolean
  Logical Operator : Logic  AllPortsSameDT=off  OutDataTypeStr=boolean
  Logical Operator1 : Logic  AllPortsSameDT=off  OutDataTypeStr=boolean
  Logical Operator2 : Logic  Operator=OR  AllPortsSameDT=off  OutDataTypeStr=boolean
  Logical Operator3 : Logic  Operator=NOT  AllPortsSameDT=off  OutDataTypeStr=boolean
  Z : Outport
  wires:
  Logical Operator2/1 -> Z/1
  I1/1 -> Data Type Conversion2/1
  Logical Operator1/1 -> Logical Operator2/2
  S/1 -> Logical Operator3/1, Logical Operator1/1
  I0/1 -> Data Type Conversion1/1
  Logical Operator/1 -> Logical Operator2/1
  Data Type Conversion1/1 -> Logical Operator/1
  Data Type Conversion2/1 -> Logical Operator1/2
  Logical Operator3/1 -> Logical Operator/2

== system labFinal_6/8-bit 4-1 MUX/4-1 MUX 2^4/2-1 MUX3 ==
  S : Inport
  I0 : Inport  Port=2
  I1 : Inport  Port=3
  Data Type Conversion1 : DataTypeConversion  OutDataTypeStr=boolean
  Data Type Conversion2 : DataTypeConversion  OutDataTypeStr=boolean
  Logical Operator : Logic  AllPortsSameDT=off  OutDataTypeStr=boolean
  Logical Operator1 : Logic  AllPortsSameDT=off  OutDataTypeStr=boolean
  Logical Operator2 : Logic  Operator=OR  AllPortsSameDT=off  OutDataTypeStr=boolean
  Logical Operator3 : Logic  Operator=NOT  AllPortsSameDT=off  OutDataTypeStr=boolean
  Z : Outport
  wires:
  Logical Operator2/1 -> Z/1
  I1/1 -> Data Type Conversion2/1
  Logical Operator1/1 -> Logical Operator2/2
  S/1 -> Logical Operator3/1, Logical Operator1/1
  I0/1 -> Data Type Conversion1/1
  Logical Operator/1 -> Logical Operator2/1
  Data Type Conversion1/1 -> Logical Operator/1
  Data Type Conversion2/1 -> Logical Operator1/2
  Logical Operator3/1 -> Logical Operator/2

== system labFinal_6/8-bit 4-1 MUX/4-1 MUX 2^4/Slicer Code ==
  uint8 : Inport  OutDataTypeStr=uint8  SampleTime=1
  Bit Slice : hdlsllib/Logic and Bit Operations/Bit Slice  lidx=0  ridx=0
  Bit Slice1 : hdlsllib/Logic and Bit Operations/Bit Slice  lidx=1  ridx=1
  Data Type Conversion : DataTypeConversion  OutDataTypeStr=boolean
  Data Type Conversion1 : DataTypeConversion  OutDataTypeStr=boolean
  S 2^1 : Outport
  "S 2^0 " : Outport  Port=2
  wires:
  Data Type Conversion1/1 -> S 2^1/1
  Data Type Conversion/1 -> "S 2^0 "/1
  Bit Slice1/1 -> Data Type Conversion1/1
  Bit Slice/1 -> Data Type Conversion/1
  uint8/1 -> Bit Slice/1, Bit Slice1/1

== system labFinal_6/8-bit 4-1 MUX/4-1 MUX 2^5/2-1 MUX1 ==
  S : Inport
  I0 : Inport  Port=2
  I1 : Inport  Port=3
  Data Type Conversion1 : DataTypeConversion  OutDataTypeStr=boolean
  Data Type Conversion2 : DataTypeConversion  OutDataTypeStr=boolean
  Logical Operator : Logic  AllPortsSameDT=off  OutDataTypeStr=boolean
  Logical Operator1 : Logic  AllPortsSameDT=off  OutDataTypeStr=boolean
  Logical Operator2 : Logic  Operator=OR  AllPortsSameDT=off  OutDataTypeStr=boolean
  Logical Operator3 : Logic  Operator=NOT  AllPortsSameDT=off  OutDataTypeStr=boolean
  Z : Outport
  wires:
  Logical Operator2/1 -> Z/1
  I1/1 -> Data Type Conversion2/1
  Logical Operator1/1 -> Logical Operator2/2
  S/1 -> Logical Operator3/1, Logical Operator1/1
  I0/1 -> Data Type Conversion1/1
  Logical Operator/1 -> Logical Operator2/1
  Data Type Conversion1/1 -> Logical Operator/1
  Data Type Conversion2/1 -> Logical Operator1/2
  Logical Operator3/1 -> Logical Operator/2

== system labFinal_6/8-bit 4-1 MUX/4-1 MUX 2^5/2-1 MUX2 ==
  S : Inport
  I0 : Inport  Port=2
  I1 : Inport  Port=3
  Data Type Conversion1 : DataTypeConversion  OutDataTypeStr=boolean
  Data Type Conversion2 : DataTypeConversion  OutDataTypeStr=boolean
  Logical Operator : Logic  AllPortsSameDT=off  OutDataTypeStr=boolean
  Logical Operator1 : Logic  AllPortsSameDT=off  OutDataTypeStr=boolean
  Logical Operator2 : Logic  Operator=OR  AllPortsSameDT=off  OutDataTypeStr=boolean
  Logical Operator3 : Logic  Operator=NOT  AllPortsSameDT=off  OutDataTypeStr=boolean
  Z : Outport
  wires:
  Logical Operator2/1 -> Z/1
  I1/1 -> Data Type Conversion2/1
  Logical Operator1/1 -> Logical Operator2/2
  S/1 -> Logical Operator3/1, Logical Operator1/1
  I0/1 -> Data Type Conversion1/1
  Logical Operator/1 -> Logical Operator2/1
  Data Type Conversion1/1 -> Logical Operator/1
  Data Type Conversion2/1 -> Logical Operator1/2
  Logical Operator3/1 -> Logical Operator/2

== system labFinal_6/8-bit 4-1 MUX/4-1 MUX 2^5/2-1 MUX3 ==
  S : Inport
  I0 : Inport  Port=2
  I1 : Inport  Port=3
  Data Type Conversion1 : DataTypeConversion  OutDataTypeStr=boolean
  Data Type Conversion2 : DataTypeConversion  OutDataTypeStr=boolean
  Logical Operator : Logic  AllPortsSameDT=off  OutDataTypeStr=boolean
  Logical Operator1 : Logic  AllPortsSameDT=off  OutDataTypeStr=boolean
  Logical Operator2 : Logic  Operator=OR  AllPortsSameDT=off  OutDataTypeStr=boolean
  Logical Operator3 : Logic  Operator=NOT  AllPortsSameDT=off  OutDataTypeStr=boolean
  Z : Outport
  wires:
  Logical Operator2/1 -> Z/1
  I1/1 -> Data Type Conversion2/1
  Logical Operator1/1 -> Logical Operator2/2
  S/1 -> Logical Operator3/1, Logical Operator1/1
  I0/1 -> Data Type Conversion1/1
  Logical Operator/1 -> Logical Operator2/1
  Data Type Conversion1/1 -> Logical Operator/1
  Data Type Conversion2/1 -> Logical Operator1/2
  Logical Operator3/1 -> Logical Operator/2

== system labFinal_6/8-bit 4-1 MUX/4-1 MUX 2^5/Slicer Code ==
  uint8 : Inport  OutDataTypeStr=uint8  SampleTime=1
  Bit Slice : hdlsllib/Logic and Bit Operations/Bit Slice  lidx=0  ridx=0
  Bit Slice1 : hdlsllib/Logic and Bit Operations/Bit Slice  lidx=1  ridx=1
  Data Type Conversion : DataTypeConversion  OutDataTypeStr=boolean
  Data Type Conversion1 : DataTypeConversion  OutDataTypeStr=boolean
  S 2^1 : Outport
  "S 2^0 " : Outport  Port=2
  wires:
  Data Type Conversion1/1 -> S 2^1/1
  Data Type Conversion/1 -> "S 2^0 "/1
  Bit Slice1/1 -> Data Type Conversion1/1
  Bit Slice/1 -> Data Type Conversion/1
  uint8/1 -> Bit Slice/1, Bit Slice1/1

== system labFinal_6/8-bit 4-1 MUX/4-1 MUX 2^6/2-1 MUX1 ==
  S : Inport
  I0 : Inport  Port=2
  I1 : Inport  Port=3
  Data Type Conversion1 : DataTypeConversion  OutDataTypeStr=boolean
  Data Type Conversion2 : DataTypeConversion  OutDataTypeStr=boolean
  Logical Operator : Logic  AllPortsSameDT=off  OutDataTypeStr=boolean
  Logical Operator1 : Logic  AllPortsSameDT=off  OutDataTypeStr=boolean
  Logical Operator2 : Logic  Operator=OR  AllPortsSameDT=off  OutDataTypeStr=boolean
  Logical Operator3 : Logic  Operator=NOT  AllPortsSameDT=off  OutDataTypeStr=boolean
  Z : Outport
  wires:
  Logical Operator2/1 -> Z/1
  I1/1 -> Data Type Conversion2/1
  Logical Operator1/1 -> Logical Operator2/2
  S/1 -> Logical Operator3/1, Logical Operator1/1
  I0/1 -> Data Type Conversion1/1
  Logical Operator/1 -> Logical Operator2/1
  Data Type Conversion1/1 -> Logical Operator/1
  Data Type Conversion2/1 -> Logical Operator1/2
  Logical Operator3/1 -> Logical Operator/2

== system labFinal_6/8-bit 4-1 MUX/4-1 MUX 2^6/2-1 MUX2 ==
  S : Inport
  I0 : Inport  Port=2
  I1 : Inport  Port=3
  Data Type Conversion1 : DataTypeConversion  OutDataTypeStr=boolean
  Data Type Conversion2 : DataTypeConversion  OutDataTypeStr=boolean
  Logical Operator : Logic  AllPortsSameDT=off  OutDataTypeStr=boolean
  Logical Operator1 : Logic  AllPortsSameDT=off  OutDataTypeStr=boolean
  Logical Operator2 : Logic  Operator=OR  AllPortsSameDT=off  OutDataTypeStr=boolean
  Logical Operator3 : Logic  Operator=NOT  AllPortsSameDT=off  OutDataTypeStr=boolean
  Z : Outport
  wires:
  Logical Operator2/1 -> Z/1
  I1/1 -> Data Type Conversion2/1
  Logical Operator1/1 -> Logical Operator2/2
  S/1 -> Logical Operator3/1, Logical Operator1/1
  I0/1 -> Data Type Conversion1/1
  Logical Operator/1 -> Logical Operator2/1
  Data Type Conversion1/1 -> Logical Operator/1
  Data Type Conversion2/1 -> Logical Operator1/2
  Logical Operator3/1 -> Logical Operator/2

== system labFinal_6/8-bit 4-1 MUX/4-1 MUX 2^6/2-1 MUX3 ==
  S : Inport
  I0 : Inport  Port=2
  I1 : Inport  Port=3
  Data Type Conversion1 : DataTypeConversion  OutDataTypeStr=boolean
  Data Type Conversion2 : DataTypeConversion  OutDataTypeStr=boolean
  Logical Operator : Logic  AllPortsSameDT=off  OutDataTypeStr=boolean
  Logical Operator1 : Logic  AllPortsSameDT=off  OutDataTypeStr=boolean
  Logical Operator2 : Logic  Operator=OR  AllPortsSameDT=off  OutDataTypeStr=boolean
  Logical Operator3 : Logic  Operator=NOT  AllPortsSameDT=off  OutDataTypeStr=boolean
  Z : Outport
  wires:
  Logical Operator2/1 -> Z/1
  I1/1 -> Data Type Conversion2/1
  Logical Operator1/1 -> Logical Operator2/2
  S/1 -> Logical Operator3/1, Logical Operator1/1
  I0/1 -> Data Type Conversion1/1
  Logical Operator/1 -> Logical Operator2/1
  Data Type Conversion1/1 -> Logical Operator/1
  Data Type Conversion2/1 -> Logical Operator1/2
  Logical Operator3/1 -> Logical Operator/2

== system labFinal_6/8-bit 4-1 MUX/4-1 MUX 2^6/Slicer Code ==
  uint8 : Inport  OutDataTypeStr=uint8  SampleTime=1
  Bit Slice : hdlsllib/Logic and Bit Operations/Bit Slice  lidx=0  ridx=0
  Bit Slice1 : hdlsllib/Logic and Bit Operations/Bit Slice  lidx=1  ridx=1
  Data Type Conversion : DataTypeConversion  OutDataTypeStr=boolean
  Data Type Conversion1 : DataTypeConversion  OutDataTypeStr=boolean
  S 2^1 : Outport
  "S 2^0 " : Outport  Port=2
  wires:
  Data Type Conversion1/1 -> S 2^1/1
  Data Type Conversion/1 -> "S 2^0 "/1
  Bit Slice1/1 -> Data Type Conversion1/1
  Bit Slice/1 -> Data Type Conversion/1
  uint8/1 -> Bit Slice/1, Bit Slice1/1

== system labFinal_6/8-bit 4-1 MUX/4-1 MUX 2^7/2-1 MUX1 ==
  S : Inport
  I0 : Inport  Port=2
  I1 : Inport  Port=3
  Data Type Conversion1 : DataTypeConversion  OutDataTypeStr=boolean
  Data Type Conversion2 : DataTypeConversion  OutDataTypeStr=boolean
  Logical Operator : Logic  AllPortsSameDT=off  OutDataTypeStr=boolean
  Logical Operator1 : Logic  AllPortsSameDT=off  OutDataTypeStr=boolean
  Logical Operator2 : Logic  Operator=OR  AllPortsSameDT=off  OutDataTypeStr=boolean
  Logical Operator3 : Logic  Operator=NOT  AllPortsSameDT=off  OutDataTypeStr=boolean
  Z : Outport
  wires:
  Logical Operator2/1 -> Z/1
  I1/1 -> Data Type Conversion2/1
  Logical Operator1/1 -> Logical Operator2/2
  S/1 -> Logical Operator3/1, Logical Operator1/1
  I0/1 -> Data Type Conversion1/1
  Logical Operator/1 -> Logical Operator2/1
  Data Type Conversion1/1 -> Logical Operator/1
  Data Type Conversion2/1 -> Logical Operator1/2
  Logical Operator3/1 -> Logical Operator/2

== system labFinal_6/8-bit 4-1 MUX/4-1 MUX 2^7/2-1 MUX2 ==
  S : Inport
  I0 : Inport  Port=2
  I1 : Inport  Port=3
  Data Type Conversion1 : DataTypeConversion  OutDataTypeStr=boolean
  Data Type Conversion2 : DataTypeConversion  OutDataTypeStr=boolean
  Logical Operator : Logic  AllPortsSameDT=off  OutDataTypeStr=boolean
  Logical Operator1 : Logic  AllPortsSameDT=off  OutDataTypeStr=boolean
  Logical Operator2 : Logic  Operator=OR  AllPortsSameDT=off  OutDataTypeStr=boolean
  Logical Operator3 : Logic  Operator=NOT  AllPortsSameDT=off  OutDataTypeStr=boolean
  Z : Outport
  wires:
  Logical Operator2/1 -> Z/1
  I1/1 -> Data Type Conversion2/1
  Logical Operator1/1 -> Logical Operator2/2
  S/1 -> Logical Operator3/1, Logical Operator1/1
  I0/1 -> Data Type Conversion1/1
  Logical Operator/1 -> Logical Operator2/1
  Data Type Conversion1/1 -> Logical Operator/1
  Data Type Conversion2/1 -> Logical Operator1/2
  Logical Operator3/1 -> Logical Operator/2

== system labFinal_6/8-bit 4-1 MUX/4-1 MUX 2^7/2-1 MUX3 ==
  S : Inport
  I0 : Inport  Port=2
  I1 : Inport  Port=3
  Data Type Conversion1 : DataTypeConversion  OutDataTypeStr=boolean
  Data Type Conversion2 : DataTypeConversion  OutDataTypeStr=boolean
  Logical Operator : Logic  AllPortsSameDT=off  OutDataTypeStr=boolean
  Logical Operator1 : Logic  AllPortsSameDT=off  OutDataTypeStr=boolean
  Logical Operator2 : Logic  Operator=OR  AllPortsSameDT=off  OutDataTypeStr=boolean
  Logical Operator3 : Logic  Operator=NOT  AllPortsSameDT=off  OutDataTypeStr=boolean
  Z : Outport
  wires:
  Logical Operator2/1 -> Z/1
  I1/1 -> Data Type Conversion2/1
  Logical Operator1/1 -> Logical Operator2/2
  S/1 -> Logical Operator3/1, Logical Operator1/1
  I0/1 -> Data Type Conversion1/1
  Logical Operator/1 -> Logical Operator2/1
  Data Type Conversion1/1 -> Logical Operator/1
  Data Type Conversion2/1 -> Logical Operator1/2
  Logical Operator3/1 -> Logical Operator/2

== system labFinal_6/8-bit 4-1 MUX/4-1 MUX 2^7/Slicer Code ==
  uint8 : Inport  OutDataTypeStr=uint8  SampleTime=1
  Bit Slice : hdlsllib/Logic and Bit Operations/Bit Slice  lidx=0  ridx=0
  Bit Slice1 : hdlsllib/Logic and Bit Operations/Bit Slice  lidx=1  ridx=1
  Data Type Conversion : DataTypeConversion  OutDataTypeStr=boolean
  Data Type Conversion1 : DataTypeConversion  OutDataTypeStr=boolean
  S 2^1 : Outport
  "S 2^0 " : Outport  Port=2
  wires:
  Data Type Conversion1/1 -> S 2^1/1
  Data Type Conversion/1 -> "S 2^0 "/1
  Bit Slice1/1 -> Data Type Conversion1/1
  Bit Slice/1 -> Data Type Conversion/1
  uint8/1 -> Bit Slice/1, Bit Slice1/1
